simulink model "Hall_Position_Estimation"  (R2025a)
settings: Solver=FixedStepDiscrete  StartTime=0.0  StopTime=10.0  FixedStep=1e-5  RelTol=1e-3
undefined symbols (not defined in the file): DiscIntNeverNeededParam
libraries: SignalEditorBlockLib x1
settings Model: Creator=86156  LastModifiedBy=86156

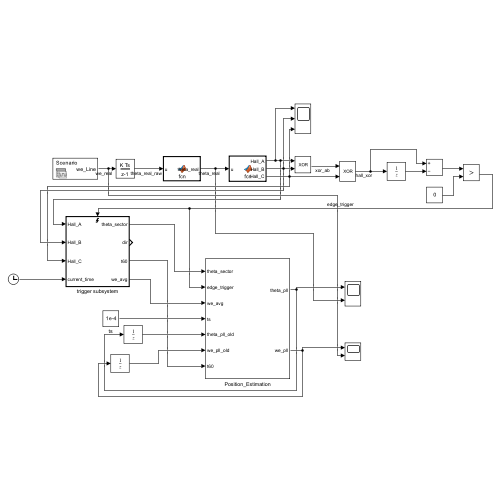
[thumbnail: Simulink's stored preview of the top-level diagram]
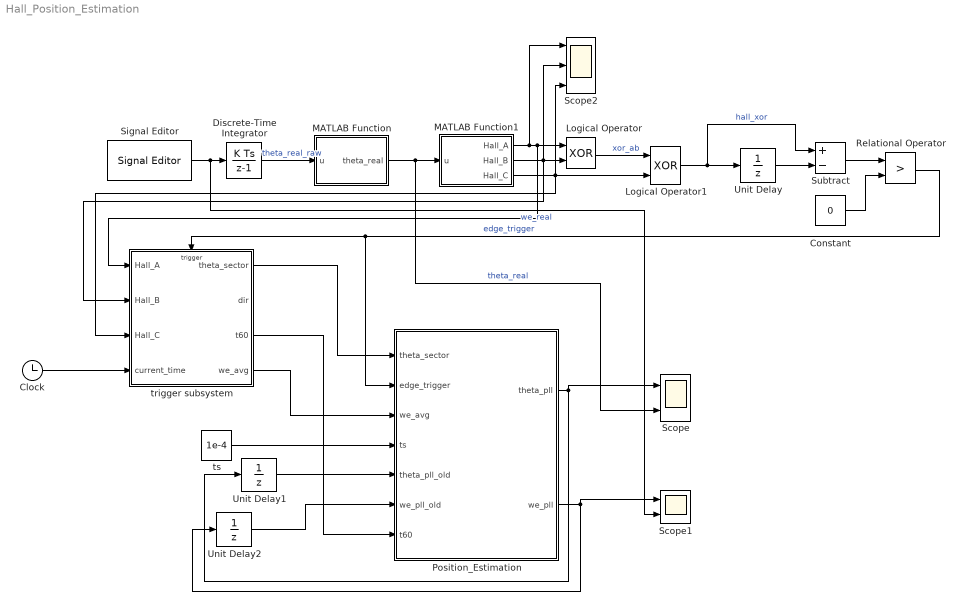
== system Hall_Position_Estimation ==
  Clock : Clock
  Constant : Constant  Value=0
  Discrete-Time Integrator : DiscreteIntegrator  SampleTime=-1  ICPrevOutput=DiscIntNeverNeededParam  ICPrevScaledInput=DiscIntNeverNeededParam
  Logical Operator : Logic  Operator=XOR  AllPortsSameDT=off  OutDataTypeStr=boolean
  Logical Operator1 : Logic  Operator=XOR  AllPortsSameDT=off  OutDataTypeStr=boolean
  MATLAB Function : MATLAB Function  TreatAsAtomicUnit=on
  MATLAB Function1 : MATLAB Function  TreatAsAtomicUnit=on
  Position_Estimation : Subsystem
  Relational Operator : RelationalOperator  Operator=>  OutDataTypeStr=boolean  RndMeth=Simplest  InputSameDT=off
  Scope : Scope  NumInputPorts=2
      settings: ActiveDisplayYMinimum=-0.785397751722092  ActiveDisplayYMaximum=7.06857976549883
  Scope1 : Scope  NumInputPorts=2
      settings: ActiveDisplayYMinimum=-28.70433653634398  ActiveDisplayYMaximum=309.47935088757532
  Scope2 : Scope  NumInputPorts=3
      settings: DataLoggingVariableName=ScopeData2
  Signal Editor : SignalEditorBlockLib/Signal Editor  FileName=D:\matlab2025a_code\model\we_line.mat  ActiveScenario=Scenario  ActiveSignal=we_Line  IsBus=off  OutputBusObjectStr=Bus: BusObject  SampleTime=0  ZeroCross=off  OutputAfterFinalValue=Setting to zero  Unit=inherit  PreserveSignalName=on  ApplySigPropsToAllScenarios=on  ApplySigPropsToAllSignals=off  SignalPropertySource=Dialog parameters
  Subtract : Sum  Inputs=+-
  Unit Delay : UnitDelay  SampleTime=-1  HasFrameUpgradeWarning=on
  Unit Delay1 : UnitDelay  SampleTime=-1  HasFrameUpgradeWarning=on
  Unit Delay2 : UnitDelay  SampleTime=-1  HasFrameUpgradeWarning=on
  trigger subsystem : Subsystem
  ts : Constant  Value=1e-4
  wires:
  Signal Editor/1 -> Scope1/2, Discrete-Time Integrator/1  "we_real"
  Discrete-Time Integrator/1 -> MATLAB Function/1(u)  "theta_real_raw"
  MATLAB Function1/1(Hall_A) -> Scope2/1, trigger subsystem/1(Hall_A), Logical Operator/1
  MATLAB Function1/2(Hall_B) -> Scope2/2, trigger subsystem/2(Hall_B), Logical Operator/2
  Logical Operator/1 -> Logical Operator1/1  "xor_ab"
  MATLAB Function1/3(Hall_C) -> trigger subsystem/3(Hall_C), Scope2/3, Logical Operator1/2
  Logical Operator1/1 -> Subtract/1, Unit Delay/1  "hall_xor"
  MATLAB Function/1(theta_real) -> Scope/2, MATLAB Function1/1(u)  "theta_real"
  Unit Delay/1 -> Subtract/2
  Subtract/1 -> Relational Operator/1
  Constant/1 -> Relational Operator/2
  Relational Operator/1 -> trigger subsystem/Trigger, Position_Estimation/2(edge_trigger)  "edge_trigger"
  Clock/1 -> trigger subsystem/4(current_time)
  trigger subsystem/1(theta_sector) -> Position_Estimation/1(theta_sector)
  trigger subsystem/4(we_avg) -> Position_Estimation/3(we_avg)
  ts/1 -> Position_Estimation/4(ts)
  Unit Delay1/1 -> Position_Estimation/5(theta_pll_old)
  Unit Delay2/1 -> Position_Estimation/6(we_pll_old)
  Position_Estimation/1(theta_pll) -> Scope/1, Unit Delay1/1
  Position_Estimation/2(we_pll) -> Scope1/1, Unit Delay2/1
  trigger subsystem/3(t60) -> Position_Estimation/7(t60)

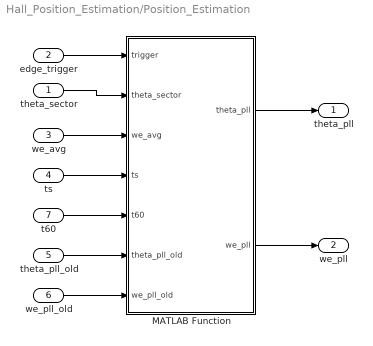
== system Hall_Position_Estimation/Position_Estimation ==
  theta_sector : Inport
  edge_trigger : Inport  Port=2
  we_avg : Inport  Port=3
  ts : Inport  Port=4
  theta_pll_old : Inport  Port=5
  we_pll_old : Inport  Port=6
  t60 : Inport  Port=7
  MATLAB Function : MATLAB Function  TreatAsAtomicUnit=on
  theta_pll : Outport
  we_pll : Outport  Port=2
  wires:
  edge_trigger/1 -> MATLAB Function/1(trigger)
  theta_sector/1 -> MATLAB Function/2(theta_sector)
  we_avg/1 -> MATLAB Function/3(we_avg)
  ts/1 -> MATLAB Function/4(ts)
  we_pll_old/1 -> MATLAB Function/7(we_pll_old)
  MATLAB Function/1(theta_pll) -> theta_pll/1
  MATLAB Function/2(we_pll) -> we_pll/1
  theta_pll_old/1 -> MATLAB Function/6(theta_pll_old)
  t60/1 -> MATLAB Function/5(t60)

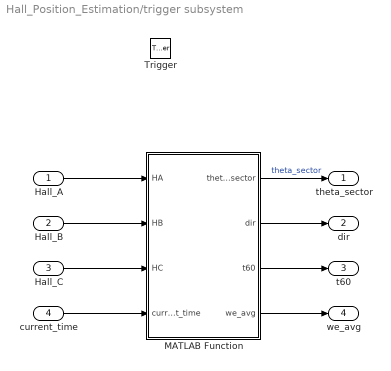
== system Hall_Position_Estimation/trigger subsystem ==
  Hall_A : Inport
  Hall_B : Inport  Port=2
  Hall_C : Inport  Port=3
  current_time : Inport  Port=4
  Trigger : TriggerPort  VariantControl=(inherit)  PortDimensions=1
  MATLAB Function : MATLAB Function  TreatAsAtomicUnit=on
  theta_sector : Outport
  dir : Outport  Port=2
  t60 : Outport  Port=3
  we_avg : Outport  Port=4
  wires:
  Hall_A/1 -> MATLAB Function/1(HA)
  Hall_B/1 -> MATLAB Function/2(HB)
  Hall_C/1 -> MATLAB Function/3(HC)
  MATLAB Function/1(theta_sector) -> theta_sector/1  "theta_sector"
  current_time/1 -> MATLAB Function/4(current_time)
  MATLAB Function/2(dir) -> dir/1
  MATLAB Function/3(t60) -> t60/1
  MATLAB Function/4(we_avg) -> we_avg/1

== matlab function Hall_Position_Estimation/MATLAB Function1 ==
  data: u input; Hall_A output; Hall_B output; Hall_C output
function [Hall_A, Hall_B, Hall_C] = fcn(u)
% 输入u是归一化后的电气角度（rad）

theta_deg = rad2deg(u);          % 转成度
theta_deg = mod(theta_deg, 360); % 归一化到[0, 360)

if (0 <= theta_deg && theta_deg < 60)
    Hall_A = 1; Hall_B = 0; Hall_C = 1;  % 扇区1 → 状态5
elseif (60 <= theta_deg && theta_deg < 120)
    Hall_A = 1; Hall_B = 0; Hall_C = 0;  % 扇区2 → 状态4
elseif (120 <= theta_deg && theta_deg < 180)
    Hall_A = 1; Hall_B = 1; Hall_C = 0;  % 扇区3 → 状态6
elseif (180 <= theta_deg && theta_deg < 240)
    Hall_A = 0; Hall_B = 1; Hall_C = 0;  % 扇区4 → 状态2
elseif (240 <= theta_deg && theta_deg < 300)
    Hall_A = 0; Hall_B = 1; Hall_C = 1;  % 扇区5 → 状态3
else
    Hall_A = 0; Hall_B = 0; Hall_C = 1;  % 扇区6 → 状态1
end
end

== matlab function Hall_Position_Estimation/MATLAB Function ==
  data: u input; theta_real output
function theta_real = fcn(u)
theta_real = mod(u, 2*pi);
if theta_real < 0
    theta_real = theta_real + 2*pi;
end
end

== matlab function Hall_Position_Estimation/trigger subsystem/MATLAB Function ==
  data: HA input; theta_sector output; HB input; HC input; current_time input; dir output; t60 output; we_avg output
function [theta_sector, dir, t60, we_avg] = fcn(HA, HB, HC, current_time)
persistent last_time last_sector buffer ptr last_we_avg
if isempty(last_time)
    last_time = 0; last_sector = 1; 
    buffer = 100*ones(6,1); ptr = 1;  % 初始用100，避免启动拉低
    last_we_avg = 100;
    theta_sector = deg2rad(30); dir = 1; t60 = 0.01; we_avg = 100;
    return;
end

% 当前扇区
state = HA*4 + HB*2 + HC;
switch state
    case 5, sector = 1; theta_sector = deg2rad(30);
    case 4, sector = 2; theta_sector = deg2rad(90);
    case 6, sector = 3; theta_sector = deg2rad(150);
    case 2, sector = 4; theta_sector = deg2rad(210);
    case 3, sector = 5; theta_sector = deg2rad(270);
    case 1, sector = 6; theta_sector = deg2rad(330);
    otherwise, sector = last_sector; theta_sector = deg2rad(30);  % 异常保持
end

% t60
t60 = current_time - last_time;
if t60 < 1e-6, t60 = 1e-6; end

% 方向（容错：大跳变当错误，保持上次dir）
delta_sector = mod(sector - last_sector + 6, 6);
if delta_sector == 1 || delta_sector == 0
    dir = 1;
elseif delta_sector == 5  % 反向正常-1
    dir = -1;
else
    dir = 1;  % 异常当正转（防噪声误反转）
end

% 瞬时速度
we_instant = (pi/3) / t60 * dir;

% 低速保护（t60>阈值或we_instant太小，保持上次平均）
if t60 > 0.05 || abs(we_instant) < 20  % 阈值可调，对应很低速
    we_avg = last_we_avg;
else
    buffer(ptr) = we_instant;
    ptr = mod(ptr,6) + 1;
    we_avg = mean(buffer);
    last_we_avg = we_avg;
end

% 更新
last_time = current_time;
last_sector = sector;
end

== matlab function Hall_Position_Estimation/Position_Estimation/MATLAB Function ==
  data: trigger input; theta_pll output; theta_sector input; we_avg input; ts input; t60 input; we_pll output; theta_pll_old input; we_pll_old input
function [theta_pll, we_pll] = fcn(trigger, theta_sector, we_avg, ts, t60, theta_pll_old, we_pll_old)
persistent kp ki max_speed low_thresh
if isempty(kp)
    kp = 500; ki = 8000; max_speed = 1500;  % 关键！kp/ki加大，响应快、低速稳
    low_thresh = 0.03;  % 低速阈值调小（您的低速t60≈0.02~0.04s）
end

% 低速直接阶梯 + 速度0（文章页6）
if t60 > low_thresh || abs(we_avg) < 60
    theta_pll = theta_sector;
    we_pll = 0;
    return;
end

% 插值（用PLL速度）
thetae_tmp = theta_pll_old;  % 初始用old
if trigger > 0.5
    thetae_tmp = theta_sector;
else
    thetae_tmp = theta_pll_old + we_pll_old * ts;
end
thetae_tmp = mod(thetae_tmp, 2*pi);

% 边界限幅
delta = thetae_tmp - theta_sector;
delta = mod(delta + pi, 2*pi) - pi;
if delta > pi/3, delta = pi/3; end
if delta < -pi/3, delta = -pi/3; end
thetae_limited = theta_sector + delta;
thetae_limited = mod(thetae_limited, 2*pi);

% PLL
err = thetae_limited - theta_pll_old;
err = mod(err + pi, 2*pi) - pi;

we_pll_new = we_pll_old + ki * err * ts;
we_pll_new = max(min(we_pll_new, max_speed), -max_speed);

theta_pll = theta_pll_old + (we_pll_new + kp * err) * ts;
theta_pll = mod(theta_pll, 2*pi);

we_pll = we_pll_new;
end
